simulink model "tripler_sps_4"  (Simulink 7.4)
settings: Solver=ode23tb  SolverMode=SingleTasking  StartTime=0.0  StopTime=.002  MaxStep=1e-6  RelTol=1e-4
PreLoadFcn:
  | Vf = .2;
StartFcn:
  | tic
StopFcn:
  | trun_sps=toc
libraries: powerlib x16, simulink x1
settings Model: MinMaxOverflowLogging=MinMaxAndOverflow  Creator=kschutz  LastModifiedBy=Dick
settings SolverCC: InitialStep=1e-9  ZeroCrossControl=EnableAll  ZeroCrossAlgorithm=Adaptive  SolverResetMethod=Robust
settings DataIOCC: SaveOutput=off  SaveTime=off
settings OptimizationCC: BooleanDataType=off  InlineParams=on  LocalBlockOutputs=off
settings DebuggingCC: AlgebraicLoopMsg=none  MaxConsecutiveZCsMsg=warning  SingleTaskRateTransMsg=error  StrictBusMsg=ErrorLevel1

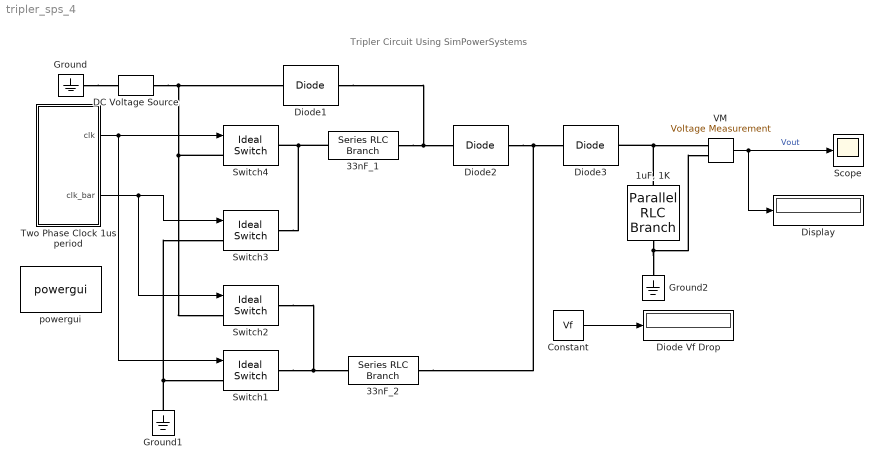
== system tripler_sps_4 ==
  note: Tripler Circuit Using SimPowerSystems
  "1uF, 1K" : powerlib/Elements/Parallel RLC Branch  DialogController=POWERSYS.PowerSysDialog  PhysicalDomain=powersysdomain  SubClassName=unknown  LeftPortType=p1  RightPortType=p1  LConnTagsString=a  RConnTagsString=__new0  BranchType=RC  Resistance=1000  Inductance=1e-3  SetiL0=off  InitialCurrent=0  Capacitance=1e-6  Setx0=off  InitialVoltage=0  Measurements=None
  33nF_1 : powerlib/Elements/Series RLC Branch  DialogController=POWERSYS.PowerSysDialog  PhysicalDomain=powersysdomain  SubClassName=unknown  LeftPortType=p1  RightPortType=p1  LConnTagsString=__new0  RConnTagsString=__new0  BranchType=C  Resistance=1  Inductance=1.0  SetiL0=off  InitialCurrent=0  Capacitance=33e-9  Setx0=off  InitialVoltage=0  Measurements=None
  33nF_2 : powerlib/Elements/Series RLC Branch  DialogController=POWERSYS.PowerSysDialog  PhysicalDomain=powersysdomain  SubClassName=unknown  LeftPortType=p1  RightPortType=p1  LConnTagsString=__new0  RConnTagsString=__new0  BranchType=C  Resistance=1  Inductance=1.0  SetiL0=off  InitialCurrent=0  Capacitance=33e-9  Setx0=off  InitialVoltage=0  Measurements=None
  Constant : Constant  Value=Vf  OutDataType=fixdt(1, 16)  OutScaling=2^0
  DC Voltage Source : powerlib/Electrical Sources/DC Voltage Source  DialogController=POWERSYS.PowerSysDialog  SystemSampleTime=-1  Amplitude=5  Measurements=None
      settings: AttributesFormatString=%<Amplitude>
  Diode Vf Drop : Display
  Diode1 : powerlib/Power Electronics/Diode  DialogController=POWERSYS.PowerSysDialog  SystemSampleTime=-1  Ron=0.001  Lon=0  Vf=Vf  IC=0  UseSnubber=off  Rs=inf  Cs=0  Measurements=off
  Diode2 : powerlib/Power Electronics/Diode  DialogController=POWERSYS.PowerSysDialog  SystemSampleTime=-1  Ron=0.001  Lon=0  Vf=Vf-.05  IC=0  UseSnubber=off  Rs=inf  Cs=0  Measurements=off
  Diode3 : powerlib/Power Electronics/Diode  DialogController=POWERSYS.PowerSysDialog  SystemSampleTime=-1  Ron=0.001  Lon=0  Vf=Vf+.025  IC=0  UseSnubber=off  Rs=inf  Cs=0  Measurements=off
  Display : Display
      settings: Decimation=100
  Ground : powerlib/Elements/Ground  DialogController=POWERSYS.PowerSysDialog  PhysicalDomain=powersysdomain  SubClassName=unknown  LeftPortType=p1  RightPortType=p1  LConnTagsString=a
  Ground1 : powerlib/Elements/Ground  DialogController=POWERSYS.PowerSysDialog  PhysicalDomain=powersysdomain  SubClassName=unknown  LeftPortType=p1  RightPortType=p1  LConnTagsString=a
  Ground2 : powerlib/Elements/Ground  DialogController=POWERSYS.PowerSysDialog  PhysicalDomain=powersysdomain  SubClassName=unknown  LeftPortType=p1  RightPortType=p1  LConnTagsString=a
  Scope : Scope
      settings: TimeRange=0.002  YMin=-1  YMax=15  MaxDataPoints=1e6  Decimation=100
  Switch1 : powerlib/Power Electronics/Ideal Switch  DialogController=POWERSYS.PowerSysDialog  SystemSampleTime=-1  Ron=10  Lon=0  IC=0  Rs=inf  Cs=inf  Measurements=off
  Switch2 : powerlib/Power Electronics/Ideal Switch  DialogController=POWERSYS.PowerSysDialog  SystemSampleTime=-1  Ron=10  Lon=0  IC=0  Rs=1e4  Cs=inf  Measurements=off
  Switch3 : powerlib/Power Electronics/Ideal Switch  DialogController=POWERSYS.PowerSysDialog  SystemSampleTime=-1  Ron=10  Lon=0  IC=0  Rs=inf  Cs=inf  Measurements=off
  Switch4 : powerlib/Power Electronics/Ideal Switch  DialogController=POWERSYS.PowerSysDialog  SystemSampleTime=-1  Ron=10  Lon=0  IC=0  Rs=1e4  Cs=inf  Measurements=off
  Two Phase Clock 1us period : Subsystem
  "VM " : powerlib/Measurements/Voltage Measurement  Tag=PoWeRsYsTeMmEaSuReMeNt  DialogController=POWERSYS.PowerSysDialog  SystemSampleTime=-1  PhasorSimulation=off  OutputType=Magnitude  PSBequivalent=0
  powergui : powerlib/powergui  Priority=1  SystemSampleTime=-1  SimulationMode=Continuous  SampleTime=50e-6  frequency=60  SPID=off  DisableSnubberDevices=on  DisableRonSwitches=on  DisableVfSwitches=on  SwTol=0  Interpol=off  frequencyindice=0  echomessages=off  HookPort=off  DisplayEquations=off  FunctionMessages=off  EnableUseOfTLC=off  x0status=blocks  RestoreLinks=warning  Frange=[0:2:500]  Ylog=off  Xlog=on  ShowGrid=off  save=off  variable=ZData  ZoomFFT=off  StartTime=0.0  cycles=1  DisplayStyle=1  fundamental=60  FreqAxis=off  MaxFrequency=1000  frequencyindicesteady=1  RmsSteady=1  display=off  Ts=0  methode=off
  wires:
  "VM "/1 -> Display/1, Scope/1  "Vout"
  Constant/1 -> Diode Vf Drop/1
  Two Phase Clock 1us period/2(clk_bar) -> Switch3/1, Switch2/1
  Two Phase Clock 1us period/1(clk) -> Switch4/1, Switch1/1
  connections:
  Ground/LConn1 -- DC Voltage Source/LConn1
  33nF_1/RConn1 -- Diode2/LConn1 -- Diode1/RConn1
  Diode2/RConn1 -- Diode3/LConn1 -- 33nF_2/RConn1
  "1uF, 1K"/LConn1 -- Diode3/RConn1 -- "VM "/LConn1
  "1uF, 1K"/RConn1 -- Ground2/LConn1 -- "VM "/LConn2
  Switch1/RConn1 -- 33nF_2/LConn1 -- Switch2/RConn1
  33nF_1/LConn1 -- Switch4/RConn1 -- Switch3/RConn1
  Ground1/LConn1 -- Switch1/LConn1 -- Switch3/LConn1
  DC Voltage Source/RConn1 -- Diode1/LConn1 -- Switch4/LConn1 -- Switch2/LConn1

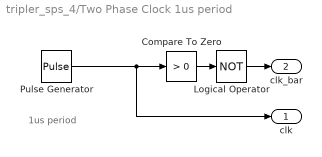
== system tripler_sps_4/Two Phase Clock 1us period ==
  note: 1us period
  Compare To Zero : simulink/Logic and Bit Operations/Compare To Zero  SystemSampleTime=-1  relop=>  LogicOutDataTypeMode=uint8
  Logical Operator : Logic  Operator=NOT  AllPortsSameDT=off  OutDataTypeMode=boolean  LogicDataType=fixdt(0, 8)  OutDataTypeStr=boolean
  Pulse Generator : DiscretePulseGenerator  PulseType=Time based  Amplitude=1  Period=1e-6  PulseWidth=50  PhaseDelay=0  SampleTime=1
  clk : Outport
  clk_bar : Outport  Port=2
  wires:
  Compare To Zero/1 -> Logical Operator/1
  Pulse Generator/1 -> Compare To Zero/1, clk/1
  Logical Operator/1 -> clk_bar/1
